simulink subsystem "ElectricalThermalSystem"  (R2024b)
settings: Solver=VariableStepAuto  StartTime=0.0  StopTime=10.0  RelTol=1e-3
undefined symbols (not defined in the file): EnvAirTemp, PlantThrEstCmpPwr, PlntThrAirBpt, PlntThrAirCond, PlntThrAirCp, PlntThrAirCpBpt, PlntThrAirPrand, PlntThrAirRho, PlntThrAirVisc, PlntThrBattDCFlwRatio, PlntThrBattJacLen, PlntThrChArea, PlntThrChDia, PlntThrCoolCond, PlntThrCoolCp, PlntThrCoolCpBpt, PlntThrCoolPrand, PlntThrCoolRho, PlntThrCoolVisc, PlntThrDCJacLen, PlntThrEMJacLen, PlntThrEstCOPLut, PlntThrEstDTLut, PlntThrHeaterMaxPwr, PlntThrPmpDisp, PlntThrPmpHeadP, PlntThrPmpMaxSpd, PlntThrPmpMechEff, PlntThrPmpVolEff, PlntThrRadAirArea, PlntThrRadAirDh, PlntThrRadFanAreaFlw, PlntThrRadFlwCoef, PlntThrRadGapHeight, PlntThrRadLength, PlntThrRadNTubes, PlntThrRadTubeDh, PlntThrRadTubeHeight, PlntThrRadWidth
libraries: autolibutils x45
(part 2 of 4)

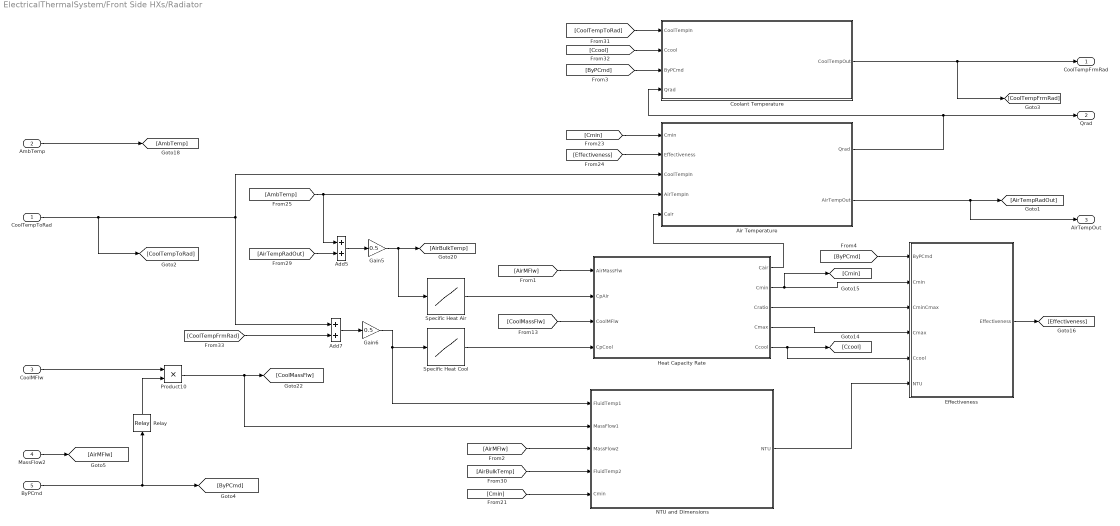
== system ElectricalThermalSystem/Front Side HXs/Radiator ==
  CoolTempToRad : Inport
  AmbTemp : Inport  Port=2
  CoolMFlw : Inport  Port=3
  MassFlow2 : Inport  Port=4
  ByPCmd : Inport  Port=5
  Add5 : Sum
  Add7 : Sum
  Air Temperature : Subsystem
      mask DialogControl DescTextVar Prompt: Air Temperature
      mask DialogControl ParameterGroupVar Prompt: Description
      mask DialogControl Control2 Prompt: Calculates the change in air temperature through the radiator and adds it to the inlet temperature to calculate the outlet temperature. In order to do that, the heat dissipated is calculated, using the effectiveness of the heat exchanger.
      mask DialogControl Control3 Prompt: Q = Effectiveness * Cmin * (Tcool - Tair)
      mask DialogControl Control4 Prompt: Where:
      mask DialogControl Control5 Prompt: Q: heat-flow rate
      mask DialogControl Control6 Prompt: Cmin: min(heat capacity rate air vs coolant)
      mask DialogControl Control7 Prompt: Heat capacity rate: heat capacity * fluid mass flow
      mask DialogControl Control8 Prompt: Tcool: coolant temperature (inlet)
      mask DialogControl Control9 Prompt: Tair: air temperature (inlet)
  Coolant Temperature : Subsystem
      mask DialogControl DescTextVar Prompt: Coolant Temperature
      mask DialogControl ParameterGroupVar Prompt: Description
      mask DialogControl Control2 Prompt: Calculates the change in coolant temperature through the radiator and adds it to the inlet temperature to calculate the outlet temperature.
      mask DialogControl Control3 Prompt: Q = Cool*(Tout-Tin)
      mask DialogControl Control4 Prompt: Where:
      mask DialogControl Control5 Prompt: Q: heat-flow rate
      mask DialogControl Control6 Prompt: Ccool (heat capacity rate) = mdot * Cp
      mask DialogControl Control7 Prompt: mdot: mass flow
      mask DialogControl Control8 Prompt: Cp: heat capacity
      mask DialogControl Control10 Prompt: Tout: temperature (outlet)
      mask DialogControl Control9 Prompt: Tin: temperature (inlet)
  Effectiveness : Subsystem
      mask DialogControl DescTextVar Prompt: Effectiveness
      mask DialogControl ParameterGroupVar Prompt: Description
      mask DialogControl Control2 Prompt: Effectiveness is calculated with NTU, according to the heat capacity rate ratio between the two fluids (air, coolant).
      mask DialogControl Control3 Prompt: If Cmax == Ccool: Effectiveness = (Cmax/Cmin)* (1-exp(-(Cmin/Cmax)*(1-exp(-NTU))))
      mask DialogControl Control4 Prompt: If Cmin == Ccool: Efectiveness = 1-exp((-Cmax/Cmin)*(1-exp(-Cmin/Cmax*NTU)))
      mask DialogControl Control5 Prompt: Where:
      mask DialogControl Control6 Prompt: Cmax: maximum heat capacity rate between the two fluids
      mask DialogControl Control7 Prompt: Cmin: minimum heat capacity rate between the two fluids
      mask DialogControl Control9 Prompt: Ccool: coolant heat capacity rate
      mask DialogControl Control8 Prompt: Heat capacity rate: heat capacity * fluid mass flow
  Gain5 : Gain  Gain=0.5
  Gain6 : Gain  Gain=0.5
  Heat Capacity Rate : Subsystem
      mask DialogControl DescTextVar Prompt: Heat Capacity Rate
      mask DialogControl ParameterGroupVar Prompt: Description
      mask DialogControl Control2 Prompt: Heat capacity rates (Cair, Ccool) are calculated for the two fluids in the heat exchanger, air and coolant.
      mask DialogControl Control3 Prompt: Cair and Ccool are used for NTU, temperature and effectiveness calculations.
      mask DialogControl Control4 Prompt: Heat capacity rate: heat capacity * fluid mass flow
  NTU and Dimensions : Subsystem  mask{NTubes=PlntThrRadNTubes, DhCool=PlntThrRadTubeDh, RadLen=PlntThrRadLength, RadWid=PlntThrRadWidth, DhAir=PlntThrRadAirDh, AcCool=PlntThrRadWidth*PlntThrRadTubeHeight, AcAir=PlntThrRadLength*PlntThrRadGapHeight*0.9}
      mask prompts: NTubes "Number of tubes, [-]"; DhCool "Hydraulic diameter coolant side, DhCool [m]"; RadLen "Radiator length, RadLen"; RadWid "Radiator width, RadWid"; DhAir "Hydraulic diameter air side, DhAir [m]"; AcCool "Cross-sectional area coolant side, AcCool [m^2]"; AcAir "Cross-sectional area air side, AcAir"
      mask TypeOptions NTubes: Constant/Value
      mask TypeOptions DhCool: Constant1/Value
      mask TypeOptions RadLen: Constant6/Value
      mask TypeOptions RadWid: Constant2/Value
      mask TypeOptions DhAir: Constant4/Value
      mask TypeOptions AcCool: Constant7/Value
      mask TypeOptions AcAir: Constant8/Value
      mask DialogControl DescTextVar Prompt: Number of Heat Transfer Units (NTU) and Radiator Dimensions
      mask DialogControl ParameterGroupVar Prompt: Description
      mask DialogControl Control1 Prompt: In heat exchangers NTU is a measure of heat transfer size.
      mask DialogControl Control3 Prompt: NTU = UA/Cmin
      mask DialogControl Control4 Prompt: Where:
      mask DialogControl Control5 Prompt: UA = 1/((1/HTCa*A)+(1/HTCc*A))
      mask DialogControl Control6 Prompt: Where:
      mask DialogControl Control7 Prompt: HTCa: convective heat transfer coefficient air side
      mask DialogControl Control8 Prompt: HTCc: convective heat transfer coefficient coolant side
      mask DialogControl Control9 Prompt: A: heat transfer area
      mask DialogControl Control10 Prompt: Cmin: min(heat capacity rate air vs coolant)
      mask DialogControl Control11 Prompt: Heat capacity rate: heat capacity * fluid mass flow
      mask DialogControl Container3 Prompt: Parameters
  Product10 : Product
  Relay : Relay  OnSwitchValue=0.5  OffSwitchValue=0.5  OnOutputValue=eps  OffOutputValue=1
  Specific Heat Air : Lookup_n-D  NumberOfTableDimensions=1  BreakpointsForDimension1=PlntThrAirCpBpt  Table=PlntThrAirCp  ExtrapMethod=Clip  UseLastTableValue=on  InternalRulePriority=Speed  RndMeth=Simplest
  Specific Heat Cool : Lookup_n-D  NumberOfTableDimensions=1  BreakpointsForDimension1=PlntThrCoolCpBpt  Table=PlntThrCoolCp  ExtrapMethod=Clip  UseLastTableValue=on  InternalRulePriority=Speed  RndMeth=Simplest
  CoolTempFrmRad : Outport
  Qrad : Outport  Port=2
  AirTempOut : Outport  Port=3
  wires:
  CoolTempToRad/1 -> Air Temperature/3(CoolTempIn), Add7/1, [CoolTempToRad]
  Gain6/1 -> NTU and Dimensions/1(FluidTemp1), Specific Heat Cool/1
  [AirBulkTemp] -> NTU and Dimensions/4(FluidTemp2)
  [CoolTempFrmRad] -> Add7/2
  CoolMFlw/1 -> Product10/1
  Product10/1 -> NTU and Dimensions/2(MassFlow1), [CoolMassFlw]
  [AmbTemp] -> Add5/1, Air Temperature/4(AirTempIn)
  ByPCmd/1 -> [ByPCmd], Relay/1
  [Cmin] -> NTU and Dimensions/5(Cmin)
  AmbTemp/1 -> [AmbTemp]
  [AirTempRadOut] -> Add5/2
  Add5/1 -> Gain5/1
  Gain5/1 -> Specific Heat Air/1, [AirBulkTemp]
  Relay/1 -> Product10/2
  Add7/1 -> Gain6/1
  MassFlow2/1 -> [AirMFlw]
  [AirMFlw] -> NTU and Dimensions/3(MassFlow2)
  Heat Capacity Rate/2(Cmin) -> Effectiveness/2(Cmin), [Cmin]
  [AirMFlw] -> Heat Capacity Rate/1(AirMassFlw)
  Specific Heat Air/1 -> Heat Capacity Rate/2(CpAir)
  [CoolMassFlw] -> Heat Capacity Rate/3(CoolMFlw)
  Specific Heat Cool/1 -> Heat Capacity Rate/4(CpCool)
  [ByPCmd] -> Effectiveness/1(ByPCmd)
  Heat Capacity Rate/3(Cratio) -> Effectiveness/3(CminCmax)
  Heat Capacity Rate/4(Cmax) -> Effectiveness/4(Cmax)
  Heat Capacity Rate/5(Ccool) -> Effectiveness/5(Ccool), [Ccool]
  NTU and Dimensions/1(NTU) -> Effectiveness/6(NTU)
  Effectiveness/1(Effectiveness) -> [Effectiveness]
  Coolant Temperature/1(CoolTempOut) -> CoolTempFrmRad/1, [CoolTempFrmRad]
  [CoolTempToRad] -> Coolant Temperature/1(CoolTempIn)
  [Ccool] -> Coolant Temperature/2(Ccool)
  Air Temperature/2(AirTempOut) -> AirTempOut/1, [AirTempRadOut]
  Air Temperature/1(Qrad) -> Coolant Temperature/4(Qrad), Qrad/1
  [Cmin] -> Air Temperature/1(Cmin)
  [Effectiveness] -> Air Temperature/2(Effectiveness)
  Heat Capacity Rate/1(Cair) -> Air Temperature/5(Cair)
  [ByPCmd] -> Coolant Temperature/3(ByPCmd)

== system ElectricalThermalSystem/Heater Battery DCDC Converter/Battery ==
  FluidTemp : Inport
  MassFlow : Inport  Port=2
  BattTemp : Inport  Port=3
  Constant3 : Constant  Value=JacHtArea  SampleTime=-1
  Constant6 : Constant  Value=JacDia  SampleTime=-1
  Constant7 : Constant  Value=JacArea  SampleTime=-1
  Constant8 : Constant  Value=JacLen  SampleTime=-1
  HTC Estimator Batt : Subsystem
      mask DialogControl Control1 Prompt: Convective Heat Transfer Coefficient (HTC) Estimator
      mask DialogControl Container2 Prompt: Description
      mask DialogControl Control2 Prompt: Assumes turbulent flow through a tube.
      mask DialogControl Control3 Prompt: The Nusselt number (NuD) is calculated with empirical formulas depending on 1/DoL.
      mask DialogControl Control4 Prompt: Where:
      mask DialogControl Control5 Prompt: DoL = hydraulic diameter / tube length
      mask DialogControl Control6 Prompt: When 1/DoL >= 400: NuD = 0.023*ReD^0.8*Pr^0.33
      mask DialogControl Control7 Prompt: Where:
      mask DialogControl Control8 Prompt: Pr: Prandtl number, out of 1D LUT depending on fluid temperature
      mask DialogControl Control9 Prompt: ReD: Reynolds number, calculated. ReD = mdot*hdia/(Ac*aVsc)
      mask DialogControl Control10 Prompt: Where:
      mask DialogControl Control11 Prompt: mdot: mass flow
      mask DialogControl Control12 Prompt: hdia: hydraulic diameter
      mask DialogControl Control13 Prompt: Ac: cross section area
      mask DialogControl Control14 Prompt: aVsc: absolute viscosity, out of 1D LUT depending on fluid temperature
      mask DialogControl Control15 Prompt: When 1/DoL < 400: NuD = 0.36*ReD^0.8*Pr^0.33*DoL^0.055
      mask DialogControl Control16 Prompt: Finally, HTC = k*NuD/hdia
      mask DialogControl Control17 Prompt: Where:
      mask DialogControl Control18 Prompt: k: thermal conductivity, out of 1D LUT depending on fluid temperature
  Heat-flow Rate : Subsystem
  Qbatt : Outport
  wires:
  Constant7/1 -> HTC Estimator Batt/3(CrossA)
  Constant8/1 -> HTC Estimator Batt/5(TubLen)
  Constant6/1 -> HTC Estimator Batt/4(HydDia)
  MassFlow/1 -> HTC Estimator Batt/2(MassFlow)
  HTC Estimator Batt/1(HTC) -> Heat-flow Rate/1(HTC)
  Constant3/1 -> Heat-flow Rate/2(JacHtArea)
  BattTemp/1 -> Heat-flow Rate/3(BattTemp)
  FluidTemp/1 -> Heat-flow Rate/4(CoolBlkTemp), HTC Estimator Batt/1(FluidTemp)
  Heat-flow Rate/1(Qbatt) -> Qbatt/1

== system ElectricalThermalSystem/Heater Battery DCDC Converter/Battery Heater ==
  HeaterCmd : Inport
  BattCoolMFlw : Inport  Port=2
  CoolTempIn : Inport  Port=3
  Add : Sum
  Add4 : Sum
  Divide1 : Product  Inputs=*/
  Gain4 : Gain  Gain=0.5
  LPF with IC3 : Subsystem  mask{wc=10, InitCond=EnvAirTemp, dataType=off}
      mask prompts: wc "Cutoff frequency, wc [rad/s]"; InitCond "Initial condition, InitCond [same as u]"; dataType "Enforce same input data type"
      mask TypeOptions wc: Cont LPF IC/wc
      mask TypeOptions InitCond: Initial Condition/Value
      mask TypeOptions dataType: Cont LPF IC/dataType
  Max Heat : Gain  Gain=HtPwr
  Product : Product
  Specific Heat1 : Lookup_n-D  NumberOfTableDimensions=1  BreakpointsForDimension1=PlntThrCoolCpBpt  Table=PlntThrCoolCp  ExtrapMethod=Clip  UseLastTableValue=on  InternalRulePriority=Speed  RndMeth=Simplest
  div0protect - abs poly1 : autolibutils/div0protect - abs poly  thresh=.001  aMode=1
  Qheater : Outport
  CoolBattTemp : Outport  Port=2
  wires:
  Gain4/1 -> Specific Heat1/1
  Divide1/1 -> Add/1
  Specific Heat1/1 -> Product/2
  Product/1 -> div0protect - abs poly1/1
  CoolTempIn/1 -> Add/2, Add4/2
  Add4/1 -> Gain4/1
  Max Heat/1 -> Qheater/1, Divide1/1
  div0protect - abs poly1/1 -> Divide1/2
  BattCoolMFlw/1 -> Product/1
  [CoolBattTempIn] -> Add4/1
  HeaterCmd/1 -> Max Heat/1
  Add/1 -> LPF with IC3/1(u)
  LPF with IC3/1(y) -> [CoolBattTempIn], CoolBattTemp/1

== system ElectricalThermalSystem/Heater Battery DCDC Converter/Coolant Mass Flow Distribution ==
  CoolMFlw : Inport
  Gain2 : Gain  Gain=MFlwRt
  Minus1 : Sum  Inputs=+-
  DCCoolMFlw : Outport
  BattCoolMFlw : Outport  Port=2
  wires:
  Gain2/1 -> BattCoolMFlw/1, Minus1/2
  CoolMFlw/1 -> Minus1/1, Gain2/1
  Minus1/1 -> DCCoolMFlw/1

== system ElectricalThermalSystem/Heater Battery DCDC Converter/Coolant Temperature ==
  Qsum : Inport
  CoolMFlw : Inport  Port=2
  CoolBlkTemp : Inport  Port=3
  Divide : Product  Inputs=*/
  Product3 : Product
  Specific Heat : Lookup_n-D  NumberOfTableDimensions=1  BreakpointsForDimension1=PlntThrCoolCpBpt  Table=PlntThrCoolCp  ExtrapMethod=Clip  UseLastTableValue=on  InternalRulePriority=Speed  RndMeth=Simplest
  div0protect - abs poly4 : autolibutils/div0protect - abs poly  thresh=.001  aMode=1
  DeltaTemp : Outport
  wires:
  Specific Heat/1 -> Product3/2
  Product3/1 -> div0protect - abs poly4/1
  div0protect - abs poly4/1 -> Divide/2
  CoolMFlw/1 -> Product3/1
  Qsum/1 -> Divide/1
  CoolBlkTemp/1 -> Specific Heat/1
  Divide/1 -> DeltaTemp/1

== system ElectricalThermalSystem/Heater Battery DCDC Converter/DC-DC Converter ==
  FluidTemp : Inport
  MassFlow : Inport  Port=2
  PwrETemp : Inport  Port=3
  Constant : Constant  Value=JacDia  SampleTime=-1
  Constant2 : Constant  Value=JacHtArea  SampleTime=-1
  Constant4 : Constant  Value=JacArea  SampleTime=-1
  Constant5 : Constant  Value=JacLen  SampleTime=-1
  HTC Estimator DCDC : Subsystem
      mask DialogControl Control1 Prompt: Convective Heat Transfer Coefficient (HTC) Estimator
      mask DialogControl Container2 Prompt: Description
      mask DialogControl Control2 Prompt: Assumes turbulent flow through a tube.
      mask DialogControl Control3 Prompt: The Nusselt number (NuD) is calculated with empirical formulas depending on 1/DoL.
      mask DialogControl Control4 Prompt: Where:
      mask DialogControl Control5 Prompt: DoL = hydraulic diameter / tube length
      mask DialogControl Control6 Prompt: When 1/DoL >= 400: NuD = 0.023*ReD^0.8*Pr^0.33
      mask DialogControl Control7 Prompt: Where:
      mask DialogControl Control8 Prompt: Pr: Prandtl number, out of 1D LUT depending on fluid temperature
      mask DialogControl Control9 Prompt: ReD: Reynolds number, calculated. ReD = mdot*hdia/(Ac*aVsc)
      mask DialogControl Control10 Prompt: Where:
      mask DialogControl Control11 Prompt: mdot: mass flow
      mask DialogControl Control12 Prompt: hdia: hydraulic diameter
      mask DialogControl Control13 Prompt: Ac: cross section area
      mask DialogControl Control14 Prompt: aVsc: absolute viscosity, out of 1D LUT depending on fluid temperature
      mask DialogControl Control15 Prompt: When 1/DoL < 400: NuD = 0.36*ReD^0.8*Pr^0.33*DoL^0.055
      mask DialogControl Control16 Prompt: Finally, HTC = k*NuD/hdia
      mask DialogControl Control17 Prompt: Where:
      mask DialogControl Control18 Prompt: k: thermal conductivity, out of 1D LUT depending on fluid temperature
  Heat-flow Rate : Subsystem
  Qpwre : Outport
  wires:
  Constant/1 -> HTC Estimator DCDC/4(HydDia)
  Constant5/1 -> HTC Estimator DCDC/5(TubLen)
  Constant4/1 -> HTC Estimator DCDC/3(CrossA)
  MassFlow/1 -> HTC Estimator DCDC/2(MassFlow)
  HTC Estimator DCDC/1(HTC) -> Heat-flow Rate/1(HTC)
  PwrETemp/1 -> Heat-flow Rate/2(PwrETemp)
  Constant2/1 -> Heat-flow Rate/3(JacArea)
  FluidTemp/1 -> Heat-flow Rate/4(CoolBlkTemp), HTC Estimator DCDC/1(FluidTemp)
  Heat-flow Rate/1(Qpwre) -> Qpwre/1

== system ElectricalThermalSystem/Heater Battery DCDC Converter/LPF with IC1 ==
  u : Inport
  Cont LPF IC : autolibutils/Cont LPF IC  wc=wc  aMode=1  dataType=off
  Initial Condition : Constant  Value=InitCond  SampleTime=-1
  y : Outport
  wires:
  Initial Condition/1 -> Cont LPF IC/2
  u/1 -> Cont LPF IC/1
  Cont LPF IC/1 -> y/1

== system ElectricalThermalSystem/Heater Battery DCDC Converter/LPF with IC2 ==
  u : Inport
  Cont LPF IC : autolibutils/Cont LPF IC  wc=wc  aMode=1  dataType=off
  Initial Condition : Constant  Value=InitCond  SampleTime=-1
  y : Outport
  wires:
  Initial Condition/1 -> Cont LPF IC/2
  u/1 -> Cont LPF IC/1
  Cont LPF IC/1 -> y/1

== system ElectricalThermalSystem/Heater Battery DCDC Converter/LPF with IC4 ==
  u : Inport
  Cont LPF IC : autolibutils/Cont LPF IC  wc=wc  aMode=1  dataType=off
  Initial Condition : Constant  Value=InitCond  SampleTime=-1
  y : Outport
  wires:
  Initial Condition/1 -> Cont LPF IC/2
  u/1 -> Cont LPF IC/1
  Cont LPF IC/1 -> y/1

== system ElectricalThermalSystem/Motor/FourEMs ==
  EMTemp : Inport
  CoolMFlow : Inport  Port=2
  CoolTempIn : Inport  Port=3
  EM1 : Subsystem  mask{JacArea=PlntThrChArea, JacDia=PlntThrChDia, JacLen=PlntThrEMJacLen, JacHtArea=PlntThrEMJacLen*pi*PlntThrChDia}
      mask prompts: JacArea "Jacket cross section area, JacArea [m^2]"; JacDia "Jacket hydraulic diameter, JacDia [m]"; JacLen "Jacket length, JacLen [m]"; JacHtArea "Jacket heat transfer area, JacHtArea [m^2]"
      mask TypeOptions JacArea: Constant2/Value
      mask TypeOptions JacDia: Constant1/Value
      mask TypeOptions JacLen: Constant3/Value
      mask TypeOptions JacHtArea: Constant/Value
      mask DialogControl DescTextVar Prompt: Electric Machine Heat Transfer
      mask DialogControl ParameterGroupVar Prompt: Description
      mask DialogControl Control2 Prompt: The cooling of the electric machine is estimated with a cooling jacket.
      mask DialogControl Container3 Prompt: Parameters
  EM2 : Subsystem  mask{JacArea=PlntThrChArea, JacDia=PlntThrChDia, JacLen=PlntThrEMJacLen, JacHtArea=PlntThrEMJacLen*pi*PlntThrChDia}
      mask prompts: JacArea "Jacket cross section area, JacArea [m^2]"; JacDia "Jacket hydraulic diameter, JacDia [m]"; JacLen "Jacket length, JacLen [m]"; JacHtArea "Jacket heat transfer area, JacHtArea [m^2]"
      mask TypeOptions JacArea: Constant2/Value
      mask TypeOptions JacDia: Constant1/Value
      mask TypeOptions JacLen: Constant3/Value
      mask TypeOptions JacHtArea: Constant/Value
      mask DialogControl DescTextVar Prompt: Electric Machine Heat Transfer
      mask DialogControl ParameterGroupVar Prompt: Description
      mask DialogControl Control2 Prompt: The cooling of the electric machine is estimated with a cooling jacket.
      mask DialogControl Container3 Prompt: Parameters
  EM3 : Subsystem  mask{JacArea=PlntThrChArea, JacDia=PlntThrChDia, JacLen=PlntThrEMJacLen, JacHtArea=PlntThrEMJacLen*pi*PlntThrChDia}
      mask prompts: JacArea "Jacket cross section area, JacArea [m^2]"; JacDia "Jacket hydraulic diameter, JacDia [m]"; JacLen "Jacket length, JacLen [m]"; JacHtArea "Jacket heat transfer area, JacHtArea [m^2]"
      mask TypeOptions JacArea: Constant2/Value
      mask TypeOptions JacDia: Constant1/Value
      mask TypeOptions JacLen: Constant3/Value
      mask TypeOptions JacHtArea: Constant/Value
      mask DialogControl DescTextVar Prompt: Electric Machine Heat Transfer
      mask DialogControl ParameterGroupVar Prompt: Description
      mask DialogControl Control2 Prompt: The cooling of the electric machine is estimated with a cooling jacket.
      mask DialogControl Container3 Prompt: Parameters
  EM4 : Subsystem  mask{JacArea=PlntThrChArea, JacDia=PlntThrChDia, JacLen=PlntThrEMJacLen, JacHtArea=PlntThrEMJacLen*pi*PlntThrChDia}
      mask prompts: JacArea "Jacket cross section area, JacArea [m^2]"; JacDia "Jacket hydraulic diameter, JacDia [m]"; JacLen "Jacket length, JacLen [m]"; JacHtArea "Jacket heat transfer area, JacHtArea [m^2]"
      mask TypeOptions JacArea: Constant2/Value
      mask TypeOptions JacDia: Constant1/Value
      mask TypeOptions JacLen: Constant3/Value
      mask TypeOptions JacHtArea: Constant/Value
      mask DialogControl DescTextVar Prompt: Electric Machine Heat Transfer
      mask DialogControl ParameterGroupVar Prompt: Description
      mask DialogControl Control2 Prompt: The cooling of the electric machine is estimated with a cooling jacket.
      mask DialogControl Container3 Prompt: Parameters
  Max of Elements : MinMax  Function=max
  Vector Concatenate : Concatenate  NumInputs=4
  Bus Element Out3 : Outport  PortName=Info  Element=Qem
  Bus Element Out1 : Outport  PortName=Info  Element=CoolTempOut
  Bus Element Out4 : Outport  PortName=Info  Element=MotorTemp
  wires:
  CoolMFlow/1 -> [MassFlow], EM1/2(CoolMFlow)
  CoolTempIn/1 -> EM1/1(CoolTempIn)
  EMTemp/1 -> Max of Elements/1, [EMTemp], EM1/3(EMTemp)
  EM1/2(CoolTempOut) -> EM2/1(CoolTempIn)
  EM1/1(Qem) -> Vector Concatenate/1
  EM2/1(Qem) -> Vector Concatenate/2
  Vector Concatenate/1 -> Bus Element Out3/1
  Max of Elements/1 -> Bus Element Out4/1
  [MassFlow] -> EM2/2(CoolMFlow)
  [EMTemp] -> EM2/3(EMTemp)
  EM2/2(CoolTempOut) -> EM3/1(CoolTempIn)
  [MassFlow] -> EM3/2(CoolMFlow)
  [EMTemp] -> EM3/3(EMTemp)
  EM3/1(Qem) -> Vector Concatenate/3
  EM4/2(CoolTempOut) -> Bus Element Out1/1
  EM3/2(CoolTempOut) -> EM4/1(CoolTempIn)
  [MassFlow] -> EM4/2(CoolMFlow)
  [EMTemp] -> EM4/3(EMTemp)
  EM4/1(Qem) -> Vector Concatenate/4

== system ElectricalThermalSystem/Motor/OneEM ==
  EMTemp : Inport
  CoolMFlow : Inport  Port=2
  CoolTempIn : Inport  Port=3
  EM1 : Subsystem  mask{JacArea=PlntThrChArea, JacDia=PlntThrChDia, JacLen=PlntThrEMJacLen, JacHtArea=PlntThrEMJacLen*pi*PlntThrChDia}
      mask prompts: JacArea "Jacket cross section area, JacArea [m^2]"; JacDia "Jacket hydraulic diameter, JacDia [m]"; JacLen "Jacket length, JacLen [m]"; JacHtArea "Jacket heat transfer area, JacHtArea [m^2]"
      mask TypeOptions JacArea: Constant2/Value
      mask TypeOptions JacDia: Constant1/Value
      mask TypeOptions JacLen: Constant3/Value
      mask TypeOptions JacHtArea: Constant/Value
      mask DialogControl DescTextVar Prompt: Electric Machine Heat Transfer
      mask DialogControl ParameterGroupVar Prompt: Description
      mask DialogControl Control2 Prompt: The cooling of the electric machine is estimated with a cooling jacket.
      mask DialogControl Container3 Prompt: Parameters
  Bus Element Out3 : Outport  PortName=Info  Element=Qem
  Bus Element Out1 : Outport  PortName=Info  Element=CoolTempOut
  Bus Element Out4 : Outport  PortName=Info  Element=MotorTemp
  wires:
  CoolMFlow/1 -> EM1/1(MassFlow)
  CoolTempIn/1 -> EM1/2(CoolTempIn)
  EM1/1(Qem) -> Bus Element Out3/1
  EMTemp/1 -> Bus Element Out4/1, EM1/3(EMTemp)
  EM1/2(CoolTempOut) -> Bus Element Out1/1

== system ElectricalThermalSystem/Motor/ThreeEMs ==
  EMTemp : Inport
  CoolMFlow : Inport  Port=2
  CoolTempIn : Inport  Port=3
  EM1 : Subsystem  mask{JacArea=PlntThrChArea, JacDia=PlntThrChDia, JacLen=PlntThrEMJacLen, JacHtArea=PlntThrEMJacLen*pi*PlntThrChDia}
      mask prompts: JacArea "Jacket cross section area, JacArea [m^2]"; JacDia "Jacket hydraulic diameter, JacDia [m]"; JacLen "Jacket length, JacLen [m]"; JacHtArea "Jacket heat transfer area, JacHtArea [m^2]"
      mask TypeOptions JacArea: Constant2/Value
      mask TypeOptions JacDia: Constant1/Value
      mask TypeOptions JacLen: Constant3/Value
      mask TypeOptions JacHtArea: Constant/Value
      mask DialogControl DescTextVar Prompt: Electric Machine Heat Transfer
      mask DialogControl ParameterGroupVar Prompt: Description
      mask DialogControl Control2 Prompt: The cooling of the electric machine is estimated with a cooling jacket.
      mask DialogControl Container3 Prompt: Parameters
  EM2 : Subsystem  mask{JacArea=PlntThrChArea, JacDia=PlntThrChDia, JacLen=PlntThrEMJacLen, JacHtArea=PlntThrEMJacLen*pi*PlntThrChDia}
      mask prompts: JacArea "Jacket cross section area, JacArea [m^2]"; JacDia "Jacket hydraulic diameter, JacDia [m]"; JacLen "Jacket length, JacLen [m]"; JacHtArea "Jacket heat transfer area, JacHtArea [m^2]"
      mask TypeOptions JacArea: Constant2/Value
      mask TypeOptions JacDia: Constant1/Value
      mask TypeOptions JacLen: Constant3/Value
      mask TypeOptions JacHtArea: Constant/Value
      mask DialogControl DescTextVar Prompt: Electric Machine Heat Transfer
      mask DialogControl ParameterGroupVar Prompt: Description
      mask DialogControl Control2 Prompt: The cooling of the electric machine is estimated with a cooling jacket.
      mask DialogControl Container3 Prompt: Parameters
  EM3 : Subsystem  mask{JacArea=PlntThrChArea, JacDia=PlntThrChDia, JacLen=PlntThrEMJacLen, JacHtArea=PlntThrEMJacLen*pi*PlntThrChDia}
      mask prompts: JacArea "Jacket cross section area, JacArea [m^2]"; JacDia "Jacket hydraulic diameter, JacDia [m]"; JacLen "Jacket length, JacLen [m]"; JacHtArea "Jacket heat transfer area, JacHtArea [m^2]"
      mask TypeOptions JacArea: Constant2/Value
      mask TypeOptions JacDia: Constant1/Value
      mask TypeOptions JacLen: Constant3/Value
      mask TypeOptions JacHtArea: Constant/Value
      mask DialogControl DescTextVar Prompt: Electric Machine Heat Transfer
      mask DialogControl ParameterGroupVar Prompt: Description
      mask DialogControl Control2 Prompt: The cooling of the electric machine is estimated with a cooling jacket.
      mask DialogControl Container3 Prompt: Parameters
  Max of Elements : MinMax  Function=max
  Vector Concatenate : Concatenate  NumInputs=3
  Bus Element Out3 : Outport  PortName=Info  Element=Qem
  Bus Element Out1 : Outport  PortName=Info  Element=CoolTempOut
  Bus Element Out4 : Outport  PortName=Info  Element=MotorTemp
  wires:
  CoolMFlow/1 -> [MassFlow], EM1/2(CoolMFlow)
  CoolTempIn/1 -> EM1/1(CoolTempIn)
  EMTemp/1 -> Max of Elements/1, [EMTemp], EM1/3(EMTemp)
  EM1/2(CoolTempOut) -> EM2/1(CoolTempIn)
  EM1/1(Qem) -> Vector Concatenate/1
  EM2/1(Qem) -> Vector Concatenate/2
  Vector Concatenate/1 -> Bus Element Out3/1
  Max of Elements/1 -> Bus Element Out4/1
  [MassFlow] -> EM2/2(CoolMFlow)
  [EMTemp] -> EM2/3(EMTemp)
  EM3/2(CoolTempOut) -> Bus Element Out1/1
  EM2/2(CoolTempOut) -> EM3/1(CoolTempIn)
  [MassFlow] -> EM3/2(CoolMFlow)
  [EMTemp] -> EM3/3(EMTemp)
  EM3/1(Qem) -> Vector Concatenate/3

== system ElectricalThermalSystem/Motor/TwoEMs ==
  EMTemp : Inport
  CoolMFlow : Inport  Port=2
  CoolTempIn : Inport  Port=3
  EM1 : Subsystem  mask{JacArea=PlntThrChArea, JacDia=PlntThrChDia, JacLen=PlntThrEMJacLen, JacHtArea=PlntThrEMJacLen*pi*PlntThrChDia}
      mask prompts: JacArea "Jacket cross section area, JacArea [m^2]"; JacDia "Jacket hydraulic diameter, JacDia [m]"; JacLen "Jacket length, JacLen [m]"; JacHtArea "Jacket heat transfer area, JacHtArea [m^2]"
      mask TypeOptions JacArea: Constant2/Value
      mask TypeOptions JacDia: Constant1/Value
      mask TypeOptions JacLen: Constant3/Value
      mask TypeOptions JacHtArea: Constant/Value
      mask DialogControl DescTextVar Prompt: Electric Machine Heat Transfer
      mask DialogControl ParameterGroupVar Prompt: Description
      mask DialogControl Control2 Prompt: The cooling of the electric machine is estimated with a cooling jacket.
      mask DialogControl Container3 Prompt: Parameters
  EM2 : Subsystem  mask{JacArea=PlntThrChArea, JacDia=PlntThrChDia, JacLen=PlntThrEMJacLen, JacHtArea=PlntThrEMJacLen*pi*PlntThrChDia}
      mask prompts: JacArea "Jacket cross section area, JacArea [m^2]"; JacDia "Jacket hydraulic diameter, JacDia [m]"; JacLen "Jacket length, JacLen [m]"; JacHtArea "Jacket heat transfer area, JacHtArea [m^2]"
      mask TypeOptions JacArea: Constant2/Value
      mask TypeOptions JacDia: Constant1/Value
      mask TypeOptions JacLen: Constant3/Value
      mask TypeOptions JacHtArea: Constant/Value
      mask DialogControl DescTextVar Prompt: Electric Machine Heat Transfer
      mask DialogControl ParameterGroupVar Prompt: Description
      mask DialogControl Control2 Prompt: The cooling of the electric machine is estimated with a cooling jacket.
      mask DialogControl Container3 Prompt: Parameters
  Max of Elements : MinMax  Function=max
  Vector Concatenate : Concatenate
  Bus Element Out3 : Outport  PortName=Info  Element=Qem
  Bus Element Out1 : Outport  PortName=Info  Element=CoolTempOut
  Bus Element Out4 : Outport  PortName=Info  Element=MotorTemp
  wires:
  CoolMFlow/1 -> [MassFlow], EM1/2(CoolMFlow)
  CoolTempIn/1 -> EM1/1(CoolTempIn)
  EMTemp/1 -> Max of Elements/1, [EMTemp], EM1/3(EMTemp)
  EM1/2(CoolTempOut) -> EM2/1(CoolTempIn)
  EM2/2(CoolTempOut) -> Bus Element Out1/1
  EM1/1(Qem) -> Vector Concatenate/1
  EM2/1(Qem) -> Vector Concatenate/2
  Vector Concatenate/1 -> Bus Element Out3/1
  Max of Elements/1 -> Bus Element Out4/1
  [MassFlow] -> EM2/2(CoolMFlow)
  [EMTemp] -> EM2/3(EMTemp)

== system ElectricalThermalSystem/Motor Pump/LPF with IC1 ==
  u : Inport
  Cont LPF IC : autolibutils/Cont LPF IC  wc=wc  aMode=1  dataType=off
  Initial Condition : Constant  Value=InitCond  SampleTime=-1
  y : Outport
  wires:
  Initial Condition/1 -> Cont LPF IC/2
  u/1 -> Cont LPF IC/1
  Cont LPF IC/1 -> y/1

== system ElectricalThermalSystem/Refrigeration Loop/Chiller Coolant Temperature ==
  Qchiller : Inport
  CoolTempOut : Inport  Port=2
  CoolTempIn : Inport  Port=3
  CoolMFlw : Inport  Port=4
  ByPCmd : Inport  Port=5
  Add : Sum
  Divide : Product  Inputs=*/
  Gain1 : Gain  Gain=0.5
  LPF with IC3 : Subsystem  mask{wc=10, InitCond=EnvAirTemp, dataType=off}
      mask prompts: wc "Cutoff frequency, wc [rad/s]"; InitCond "Initial condition, InitCond [same as u]"; dataType "Enforce same input data type"
      mask TypeOptions wc: Cont LPF IC/wc
      mask TypeOptions InitCond: Initial Condition/Value
      mask TypeOptions dataType: Cont LPF IC/dataType
  Minus : Sum
  Product : Product
  Specific Heat : Lookup_n-D  NumberOfTableDimensions=1  BreakpointsForDimension1=PlntThrCoolCpBpt  Table=PlntThrCoolCp  ExtrapMethod=Clip  UseLastTableValue=on  InternalRulePriority=Speed  RndMeth=Simplest
  Switch6 : Switch  Criteria=u2 > Threshold  Threshold=0.5  SaturateOnIntegerOverflow=off  InputSameDT=off
  div0protect - abs poly2 : autolibutils/div0protect - abs poly  thresh=.001  aMode=1
  CoolTOut : Outport
  wires:
  Divide/1 -> Minus/2
  CoolTempIn/1 -> Add/2, [CoolTempIn]
  Add/1 -> Gain1/1
  Minus/1 -> LPF with IC3/1(u)
  LPF with IC3/1(y) -> Switch6/3
  [CoolTempIn] -> Minus/1, Switch6/1
  div0protect - abs poly2/1 -> Divide/2
  Gain1/1 -> Specific Heat/1
  ByPCmd/1 -> Switch6/2
  Specific Heat/1 -> Product/1
  Product/1 -> div0protect - abs poly2/1
  CoolTempOut/1 -> Add/1
  Switch6/1 -> CoolTOut/1
  Qchiller/1 -> Divide/1
  CoolMFlw/1 -> Product/2

== system ElectricalThermalSystem/Refrigeration Loop/Chiller Pressure ==
  CoolTempIn : Inport
  CoolTempOut : Inport  Port=2
  1-D Lookup Table2 : Lookup_n-D  NumberOfTableDimensions=1  BreakpointsForDimension1=[0 1 3 7]  Table=[0.65 0.45 0.3 0.3]  ExtrapMethod=Clip  UseLastTableValue=on  InternalRulePriority=Speed  RndMeth=Simplest
  Subtract3 : Sum  Inputs=+-
  ChlrPress : Outport
  wires:
  Subtract3/1 -> 1-D Lookup Table2/1
  CoolTempIn/1 -> Subtract3/1
  CoolTempOut/1 -> Subtract3/2
  1-D Lookup Table2/1 -> ChlrPress/1

== system ElectricalThermalSystem/Refrigeration Loop/Condenser Pressure ==
  AirTempOut : Inport
  AirTempIn : Inport  Port=2
  1-D Lookup Table1 : Lookup_n-D  NumberOfTableDimensions=1  BreakpointsForDimension1=[0 4.5 10 13 20]  Table=[1.3 1.3 1.53 1.62 1.7]  ExtrapMethod=Clip  UseLastTableValue=on  InternalRulePriority=Speed  RndMeth=Simplest
  Subtract1 : Sum  Inputs=+-
  CondPress : Outport
  wires:
  Subtract1/1 -> 1-D Lookup Table1/1
  AirTempOut/1 -> Subtract1/1
  AirTempIn/1 -> Subtract1/2
  1-D Lookup Table1/1 -> CondPress/1

== system ElectricalThermalSystem/Refrigeration Loop/Heat-flow Rate and Power ==
  AmbTemp : Inport
  CoolTempIn : Inport  Port=2
  CmpCmd : Inport  Port=3
  1-D Lookup Table : Lookup_n-D  NumberOfTableDimensions=1  BreakpointsForDimension1=PlntThrEstDTLut  Table=PlntThrEstCOPLut  ExtrapMethod=Clip  InternalRulePriority=Speed  RndMeth=Simplest
  Add1 : Sum
  Gain : Gain  Gain=-1
  LPF with IC1 : Subsystem  mask{wc=0.2, InitCond=0, dataType=off}
      mask prompts: wc "Cutoff frequency, wc [rad/s]"; InitCond "Initial condition, InitCond [same as u]"; dataType "Enforce same input data type"
      mask TypeOptions wc: Cont LPF IC/wc
      mask TypeOptions InitCond: Initial Condition/Value
      mask TypeOptions dataType: Cont LPF IC/dataType
  Power Chiller : Product
  Power Comp : Gain  Gain=PlantThrEstCmpPwr
  Signal Specification : SignalSpecification  Unit=kW
  Signal Specification1 : SignalSpecification  Unit=watt
  Subtract : Sum  Inputs=+-
  Unit Conversion : UnitConversion
  Qcond : Outport
  CmpPwr : Outport  Port=2
  Qchiller : Outport  Port=3
  wires:
  Unit Conversion/1 -> Signal Specification1/1
  CoolTempIn/1 -> Subtract/2
  1-D Lookup Table/1 -> Power Chiller/1
  LPF with IC1/1(y) -> Power Comp/1
  [CmpPwr] -> Add1/1
  Subtract/1 -> 1-D Lookup Table/1
  Power Chiller/1 -> Add1/2, Gain/1
  Signal Specification/1 -> Unit Conversion/1
  Power Comp/1 -> Signal Specification/1
  Signal Specification1/1 -> CmpPwr/1, [CmpPwr], Power Chiller/2
  AmbTemp/1 -> Subtract/1
  Add1/1 -> Qcond/1
  Gain/1 -> Qchiller/1
  CmpCmd/1 -> LPF with IC1/1(u)

== system ElectricalThermalSystem/Front Side HXs/Condenser/LPF with IC2 ==
  u : Inport
  Cont LPF IC : autolibutils/Cont LPF IC  wc=wc  aMode=1  dataType=off
  Initial Condition : Constant  Value=InitCond  SampleTime=-1
  y : Outport
  wires:
  Initial Condition/1 -> Cont LPF IC/2
  u/1 -> Cont LPF IC/1
  Cont LPF IC/1 -> y/1

== system ElectricalThermalSystem/Front Side HXs/Radiator/Air Temperature ==
  Cmin : Inport
  Effectiveness : Inport  Port=2
  CoolTempIn : Inport  Port=3
  AirTempIn : Inport  Port=4
  Cair : Inport  Port=5
  Add4 : Sum
  LPF with IC1 : Subsystem  mask{wc=10, InitCond=EnvAirTemp, dataType=off}
      mask prompts: wc "Cutoff frequency, wc [rad/s]"; InitCond "Initial condition, InitCond [same as u]"; dataType "Enforce same input data type"
      mask TypeOptions wc: Cont LPF IC/wc
      mask TypeOptions InitCond: Initial Condition/Value
      mask TypeOptions dataType: Cont LPF IC/dataType
  Product3 : Product  Inputs=3
  Product5 : Product  Inputs=*/
  Saturation1 : Saturate  UpperLimit=inf  LowerLimit=173.15
  Subtract : Sum  Inputs=+-
  div0protect - abs poly1 : autolibutils/div0protect - abs poly  thresh=.001  aMode=1
  Qrad : Outport
  AirTempOut : Outport  Port=2
  wires:
  Subtract/1 -> Product3/3
  Cair/1 -> div0protect - abs poly1/1
  Add4/1 -> Saturation1/1
  Saturation1/1 -> LPF with IC1/1(u)
  div0protect - abs poly1/1 -> Product5/2
  Product3/1 -> Qrad/1, Product5/1
  LPF with IC1/1(y) -> AirTempOut/1
  Product5/1 -> Add4/2
  Cmin/1 -> Product3/1
  CoolTempIn/1 -> Subtract/1
  Effectiveness/1 -> Product3/2
  AirTempIn/1 -> [AirTempIn], Subtract/2
  [AirTempIn] -> Add4/1

== system ElectricalThermalSystem/Front Side HXs/Radiator/Coolant Temperature ==
  CoolTempIn : Inport
  Ccool : Inport  Port=2
  ByPCmd : Inport  Port=3
  Qrad : Inport  Port=4
  Add6 : Sum  Inputs=+-
  LPF Temperature : Subsystem  mask{wc=1, InitCond=EnvAirTemp, dataType=off}
      mask prompts: wc "Cutoff frequency, wc [rad/s]"; InitCond "Initial condition, InitCond [same as u]"; dataType "Enforce same input data type"
      mask TypeOptions wc: Cont LPF IC/wc
      mask TypeOptions InitCond: Initial Condition/Value
      mask TypeOptions dataType: Cont LPF IC/dataType
  Product6 : Product  Inputs=*/
  Saturation : Saturate  UpperLimit=inf  LowerLimit=173.15
  Switch5 : Switch  Criteria=u2 > Threshold  Threshold=0.5  SaturateOnIntegerOverflow=off  InputSameDT=off
  div0protect - abs poly : autolibutils/div0protect - abs poly  thresh=.001  aMode=1
  CoolTempOut : Outport
  wires:
  ByPCmd/1 -> Switch5/2
  Add6/1 -> Saturation/1
  Switch5/1 -> LPF Temperature/1(u)
  LPF Temperature/1(y) -> CoolTempOut/1
  Product6/1 -> Add6/2
  CoolTempIn/1 -> Add6/1, Switch5/1
  div0protect - abs poly/1 -> Product6/2
  Saturation/1 -> Switch5/3
  Qrad/1 -> Product6/1
  Ccool/1 -> div0protect - abs poly/1

== system ElectricalThermalSystem/Front Side HXs/Radiator/Effectiveness ==
  ByPCmd : Inport
  Cmin : Inport  Port=2
  CminCmax : Inport  Port=3
  Cmax : Inport  Port=4
  Ccool : Inport  Port=5
  NTU : Inport  Port=6
  Constant5 : Constant  SampleTime=-1
  Constant9 : Constant  Value=0  SampleTime=-1
  Effectiveness Calc : Fcn  Expr=(u(3)==u(5))*(1/u(2))*(1-exp(-u(2)*(1-exp(-u(4)))))+(u(1)==u(5))*(1-exp((-1/u(2))*(1-exp(-u(2)*u(4)))))
  Product2 : Product
  Switch1 : Switch  Criteria=u2 > Threshold  Threshold=0.5  SaturateOnIntegerOverflow=off  InputSameDT=off
  Vector Concatenate : Concatenate  NumInputs=5
  div0protect - abs poly5 : autolibutils/div0protect - abs poly  thresh=.001  aMode=1
  Effectiveness : Outport
  wires:
  Switch1/1 -> Product2/1
  Constant5/1 -> Switch1/3
  Constant9/1 -> Switch1/1
  Product2/1 -> Effectiveness/1
  Effectiveness Calc/1 -> Product2/2
  Cmax/1 -> Vector Concatenate/3
  Vector Concatenate/1 -> Effectiveness Calc/1
  Cmin/1 -> Vector Concatenate/1
  Ccool/1 -> Vector Concatenate/5
  ByPCmd/1 -> Switch1/2
  NTU/1 -> Vector Concatenate/4
  div0protect - abs poly5/1 -> Vector Concatenate/2
  CminCmax/1 -> div0protect - abs poly5/1

== system ElectricalThermalSystem/Front Side HXs/Radiator/Heat Capacity Rate ==
  AirMassFlw : Inport
  CpAir : Inport  Port=2
  CoolMFlw : Inport  Port=3
  CpCool : Inport  Port=4
  Divide2 : Product  Inputs=*/  RndMeth=Zero  SaturateOnIntegerOverflow=on
  Min : MinMax  Function=max  Inputs=2
  Min1 : MinMax  Inputs=2
  Product : Product
  Product1 : Product
  div0protect - abs poly2 : autolibutils/div0protect - abs poly  thresh=.001  aMode=1
  Cair : Outport
  Cmin : Outport  Port=2
  Cratio : Outport  Port=3
  Cmax : Outport  Port=4
  Ccool : Outport  Port=5
  wires:
  Product1/1 -> Ccool/1, [Ccool], Min/2
  [Ccool] -> Min1/2  "Ccool"
  Min/1 -> Cmax/1, div0protect - abs poly2/1  "Cmax"
  CpAir/1 -> Product/2
  Min1/1 -> Cmin/1, Divide2/1
  div0protect - abs poly2/1 -> Divide2/2
  Product/1 -> Cair/1, Min1/1, Min/1
  Divide2/1 -> Cratio/1
  CpCool/1 -> Product1/2
  AirMassFlw/1 -> Product/1
  CoolMFlw/1 -> Product1/1

== system ElectricalThermalSystem/Front Side HXs/Radiator/NTU and Dimensions ==
  FluidTemp1 : Inport
  MassFlow1 : Inport  Port=2
  MassFlow2 : Inport  Port=3
  FluidTemp2 : Inport  Port=4
  Cmin : Inport  Port=5
  Add : Sum
  Bias : Bias  Bias=1  SaturateOnIntegerOverflow=off
  Constant : Constant  Value=NTubes  SampleTime=-1
  Constant1 : Constant  Value=DhCool  SampleTime=-1
  Constant2 : Constant  Value=RadWid  SampleTime=-1
  Constant4 : Constant  Value=DhAir  SampleTime=-1
  Constant6 : Constant  Value=RadLen  SampleTime=-1
  Constant7 : Constant  Value=AcCool  SampleTime=-1
  Constant8 : Constant  Value=AcAir  SampleTime=-1
  Divide : Product  Inputs=*/
  Divide1 : Product  Inputs=*/
  Divide3 : Product  Inputs=*/
  Gain : Gain  Gain=PlntThrRadAirArea
  Gain1 : Gain  Gain=PlntThrRadAirArea
  HTC Estimator Air : Subsystem
      mask DialogControl Control1 Prompt: Convective Heat Transfer Coefficient (HTC) Estimator
      mask DialogControl Container2 Prompt: Description
      mask DialogControl Control2 Prompt: Assumes turbulent flow through a tube.
      mask DialogControl Control3 Prompt: The Nusselt number (NuD) is calculated with empirical formulas depending on 1/DoL.
      mask DialogControl Control4 Prompt: Where:
      mask DialogControl Control5 Prompt: DoL = hydraulic diameter / tube length
      mask DialogControl Control6 Prompt: When 1/DoL >= 400: NuD = 0.023*ReD^0.8*Pr^0.33
      mask DialogControl Control7 Prompt: Where:
      mask DialogControl Control8 Prompt: Pr: Prandtl number, out of 1D LUT depending on fluid temperature
      mask DialogControl Control9 Prompt: ReD: Reynolds number, calculated. ReD = mdot*hdia/(Ac*aVsc)
      mask DialogControl Control10 Prompt: Where:
      mask DialogControl Control11 Prompt: mdot: mass flow
      mask DialogControl Control12 Prompt: hdia: hydraulic diameter
      mask DialogControl Control13 Prompt: Ac: cross section area
      mask DialogControl Control14 Prompt: aVsc: absolute viscosity, out of 1D LUT depending on fluid temperature
      mask DialogControl Control15 Prompt: When 1/DoL < 400: NuD = 0.36*ReD^0.8*Pr^0.33*DoL^0.055
      mask DialogControl Control16 Prompt: Finally, HTC = k*NuD/hdia
      mask DialogControl Control17 Prompt: Where:
      mask DialogControl Control18 Prompt: k: thermal conductivity, out of 1D LUT depending on fluid temperature
  HTC Estimator Coolant : Subsystem
      mask DialogControl Control1 Prompt: Convective Heat Transfer Coefficient (HTC) Estimator
      mask DialogControl Container2 Prompt: Description
      mask DialogControl Control2 Prompt: Assumes turbulent flow through a tube.
      mask DialogControl Control3 Prompt: The Nusselt number (NuD) is calculated with empirical formulas depending on 1/DoL.
      mask DialogControl Control4 Prompt: Where:
      mask DialogControl Control5 Prompt: DoL = hydraulic diameter / tube length
      mask DialogControl Control6 Prompt: When 1/DoL >= 400: NuD = 0.023*ReD^0.8*Pr^0.33
      mask DialogControl Control7 Prompt: Where:
      mask DialogControl Control8 Prompt: Pr: Prandtl number, out of 1D LUT depending on fluid temperature
      mask DialogControl Control9 Prompt: ReD: Reynolds number, calculated. ReD = mdot*hdia/(Ac*aVsc)
      mask DialogControl Control10 Prompt: Where:
      mask DialogControl Control11 Prompt: mdot: mass flow
      mask DialogControl Control12 Prompt: hdia: hydraulic diameter
      mask DialogControl Control13 Prompt: Ac: cross section area
      mask DialogControl Control14 Prompt: aVsc: absolute viscosity, out of 1D LUT depending on fluid temperature
      mask DialogControl Control15 Prompt: When 1/DoL < 400: NuD = 0.36*ReD^0.8*Pr^0.33*DoL^0.055
      mask DialogControl Control16 Prompt: Finally, HTC = k*NuD/hdia
      mask DialogControl Control17 Prompt: Where:
      mask DialogControl Control18 Prompt: k: thermal conductivity, out of 1D LUT depending on fluid temperature
  Math Function : Math  Operator=reciprocal
  Math Function1 : Math  Operator=reciprocal
  Math Function2 : Math  Operator=reciprocal
  div0protect - abs poly{1..5} (5 alike) : autolibutils/div0protect - abs poly  thresh=.001  aMode=1
  NTU : Outport
  wires:
  Constant2/1 -> HTC Estimator Air/5(TubLen)
  HTC Estimator Coolant/1(HTC) -> Gain/1
  Constant6/1 -> HTC Estimator Coolant/5(TubLen)
  Constant/1 -> div0protect - abs poly1/1, Bias/1
  MassFlow1/1 -> Divide/1
  Bias/1 -> Divide1/2
  FluidTemp2/1 -> HTC Estimator Air/1(FluidTemp)
  Divide/1 -> HTC Estimator Coolant/2(MassFlow)
  FluidTemp1/1 -> HTC Estimator Coolant/1(FluidTemp)
  Constant7/1 -> HTC Estimator Coolant/3(CrossA)
  Divide1/1 -> HTC Estimator Air/2(MassFlow)
  Constant8/1 -> HTC Estimator Air/3(CrossA)
  HTC Estimator Air/1(HTC) -> Gain1/1
  Constant1/1 -> HTC Estimator Coolant/4(HydDia)
  Constant4/1 -> HTC Estimator Air/4(HydDia)
  MassFlow2/1 -> Divide1/1
  Divide3/1 -> NTU/1
  div0protect - abs poly3/1 -> Divide3/2
  Cmin/1 -> div0protect - abs poly3/1
  div0protect - abs poly1/1 -> Divide/2
  Math Function2/1 -> Divide3/1
  div0protect - abs poly5/1 -> Math Function2/1
  Add/1 -> div0protect - abs poly5/1
  div0protect - abs poly4/1 -> Math Function1/1
  Gain1/1 -> div0protect - abs poly4/1
  Gain/1 -> div0protect - abs poly2/1
  div0protect - abs poly2/1 -> Math Function/1
  Math Function/1 -> Add/1
  Math Function1/1 -> Add/2

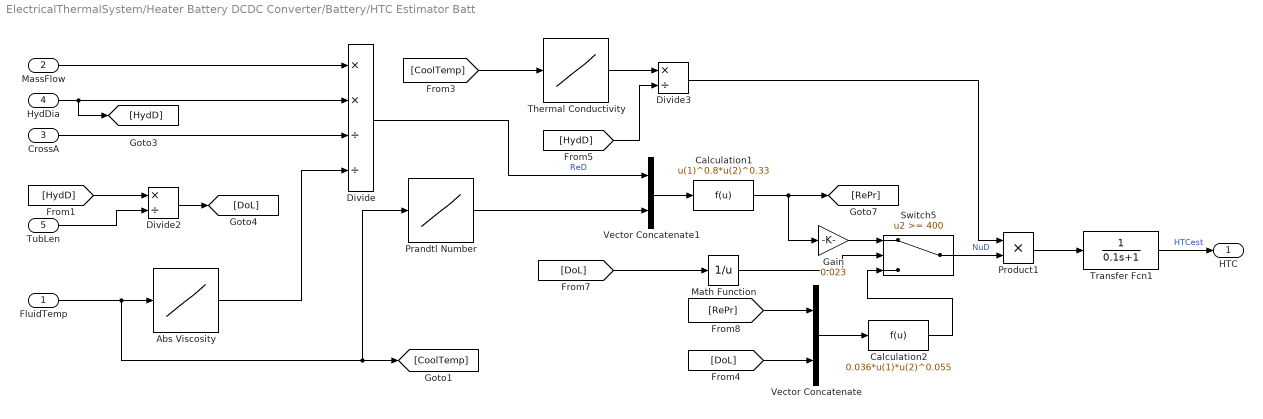
== system ElectricalThermalSystem/Heater Battery DCDC Converter/Battery/HTC Estimator Batt ==
  FluidTemp : Inport
  MassFlow : Inport  Port=2
  CrossA : Inport  Port=3  OutMin=eps
  HydDia : Inport  Port=4
  TubLen : Inport  Port=5
  Abs Viscosity : Lookup_n-D  NumberOfTableDimensions=1  BreakpointsForDimension1=PlntThrCoolCpBpt  Table=PlntThrCoolVisc  ExtrapMethod=Clip  UseLastTableValue=on  InternalRulePriority=Speed  RndMeth=Simplest
  Calculation1 : Fcn  Expr=u(1)^0.8*u(2)^0.33
  Calculation2 : Fcn  Expr=0.036*u(1)*u(2)^0.055
  Divide : Product  Inputs=**//
  Divide2 : Product  Inputs=*/
  Divide3 : Product  Inputs=*/
  Gain : Gain  Gain=0.023
  Math Function : Math  Operator=reciprocal
  Prandtl Number : Lookup_n-D  NumberOfTableDimensions=1  BreakpointsForDimension1=PlntThrCoolCpBpt  Table=PlntThrCoolPrand  ExtrapMethod=Clip  UseLastTableValue=on  InternalRulePriority=Speed  RndMeth=Simplest
  Product1 : Product
  Switch5 : Switch  Threshold=400  SaturateOnIntegerOverflow=off  InputSameDT=off
  Thermal Conductivity : Lookup_n-D  NumberOfTableDimensions=1  BreakpointsForDimension1=PlntThrCoolCpBpt  Table=PlntThrCoolCond  ExtrapMethod=Clip  UseLastTableValue=on  InternalRulePriority=Speed  RndMeth=Simplest
  Transfer Fcn1 : TransferFcn  Denominator=[0.1 1]
  Vector Concatenate : Concatenate
  Vector Concatenate1 : Concatenate
  HTC : Outport
  wires:
  Transfer Fcn1/1 -> HTC/1  "HTCest"
  FluidTemp/1 -> Prandtl Number/1, [CoolTemp], Abs Viscosity/1
  [CoolTemp] -> Thermal Conductivity/1
  MassFlow/1 -> Divide/1
  HydDia/1 -> [HydD], Divide/2
  CrossA/1 -> Divide/3
  [HydD] -> Divide2/1
  TubLen/1 -> Divide2/2
  Divide2/1 -> [DoL]
  Abs Viscosity/1 -> Divide/4
  Divide/1 -> Vector Concatenate1/1  "ReD"
  Prandtl Number/1 -> Vector Concatenate1/2
  Vector Concatenate1/1 -> Calculation1/1
  [DoL] -> Math Function/1
  Math Function/1 -> Switch5/2
  Thermal Conductivity/1 -> Divide3/1
  [HydD] -> Divide3/2
  Divide3/1 -> Product1/1
  Gain/1 -> Switch5/1
  Calculation1/1 -> [RePr], Gain/1
  [RePr] -> Vector Concatenate/1
  [DoL] -> Vector Concatenate/2
  Vector Concatenate/1 -> Calculation2/1
  Calculation2/1 -> Switch5/3
  Switch5/1 -> Product1/2  "NuD"
  Product1/1 -> Transfer Fcn1/1

== system ElectricalThermalSystem/Heater Battery DCDC Converter/Battery/Heat-flow Rate ==
  HTC : Inport
  JacHtArea : Inport  Port=2
  BattTemp : Inport  Port=3
  CoolBlkTemp : Inport  Port=4
  Product2 : Product  Inputs=3
  Subtract1 : Sum  Inputs=+-
  Qbatt : Outport
  wires:
  HTC/1 -> Product2/1
  Subtract1/1 -> Product2/3
  JacHtArea/1 -> Product2/2
  CoolBlkTemp/1 -> Subtract1/2
  Product2/1 -> Qbatt/1
  BattTemp/1 -> Subtract1/1

== system ElectricalThermalSystem/Heater Battery DCDC Converter/Battery Heater/LPF with IC3 ==
  u : Inport
  Cont LPF IC : autolibutils/Cont LPF IC  wc=wc  aMode=1  dataType=off
  Initial Condition : Constant  Value=InitCond  SampleTime=-1
  y : Outport
  wires:
  Initial Condition/1 -> Cont LPF IC/2
  u/1 -> Cont LPF IC/1
  Cont LPF IC/1 -> y/1

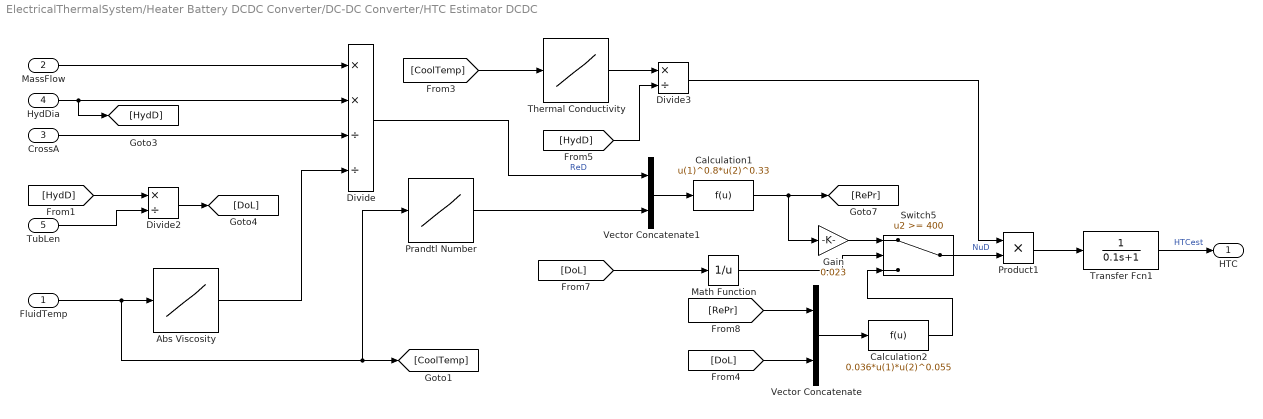
== system ElectricalThermalSystem/Heater Battery DCDC Converter/DC-DC Converter/HTC Estimator DCDC ==
  FluidTemp : Inport
  MassFlow : Inport  Port=2
  CrossA : Inport  Port=3  OutMin=eps
  HydDia : Inport  Port=4
  TubLen : Inport  Port=5
  Abs Viscosity : Lookup_n-D  NumberOfTableDimensions=1  BreakpointsForDimension1=PlntThrCoolCpBpt  Table=PlntThrCoolVisc  ExtrapMethod=Clip  UseLastTableValue=on  InternalRulePriority=Speed  RndMeth=Simplest
  Calculation1 : Fcn  Expr=u(1)^0.8*u(2)^0.33
  Calculation2 : Fcn  Expr=0.036*u(1)*u(2)^0.055
  Divide : Product  Inputs=**//
  Divide2 : Product  Inputs=*/
  Divide3 : Product  Inputs=*/
  Gain : Gain  Gain=0.023
  Math Function : Math  Operator=reciprocal
  Prandtl Number : Lookup_n-D  NumberOfTableDimensions=1  BreakpointsForDimension1=PlntThrCoolCpBpt  Table=PlntThrCoolPrand  ExtrapMethod=Clip  UseLastTableValue=on  InternalRulePriority=Speed  RndMeth=Simplest
  Product1 : Product
  Switch5 : Switch  Threshold=400  SaturateOnIntegerOverflow=off  InputSameDT=off
  Thermal Conductivity : Lookup_n-D  NumberOfTableDimensions=1  BreakpointsForDimension1=PlntThrCoolCpBpt  Table=PlntThrCoolCond  ExtrapMethod=Clip  UseLastTableValue=on  InternalRulePriority=Speed  RndMeth=Simplest
  Transfer Fcn1 : TransferFcn  Denominator=[0.1 1]
  Vector Concatenate : Concatenate
  Vector Concatenate1 : Concatenate
  HTC : Outport
  wires:
  Transfer Fcn1/1 -> HTC/1  "HTCest"
  FluidTemp/1 -> Prandtl Number/1, [CoolTemp], Abs Viscosity/1
  [CoolTemp] -> Thermal Conductivity/1
  MassFlow/1 -> Divide/1
  HydDia/1 -> [HydD], Divide/2
  CrossA/1 -> Divide/3
  [HydD] -> Divide2/1
  TubLen/1 -> Divide2/2
  Divide2/1 -> [DoL]
  Abs Viscosity/1 -> Divide/4
  Divide/1 -> Vector Concatenate1/1  "ReD"
  Prandtl Number/1 -> Vector Concatenate1/2
  Vector Concatenate1/1 -> Calculation1/1
  [DoL] -> Math Function/1
  Math Function/1 -> Switch5/2
  Thermal Conductivity/1 -> Divide3/1
  [HydD] -> Divide3/2
  Divide3/1 -> Product1/1
  Gain/1 -> Switch5/1
  Calculation1/1 -> [RePr], Gain/1
  [RePr] -> Vector Concatenate/1
  [DoL] -> Vector Concatenate/2
  Vector Concatenate/1 -> Calculation2/1
  Calculation2/1 -> Switch5/3
  Switch5/1 -> Product1/2  "NuD"
  Product1/1 -> Transfer Fcn1/1

== system ElectricalThermalSystem/Heater Battery DCDC Converter/DC-DC Converter/Heat-flow Rate ==
  HTC : Inport
  PwrETemp : Inport  Port=2
  JacArea : Inport  Port=3
  CoolBlkTemp : Inport  Port=4
  Product1 : Product  Inputs=3
  Subtract : Sum  Inputs=+-
  Qpwre : Outport
  wires:
  JacArea/1 -> Product1/2
  Subtract/1 -> Product1/3
  PwrETemp/1 -> Subtract/1
  CoolBlkTemp/1 -> Subtract/2
  Product1/1 -> Qpwre/1
  HTC/1 -> Product1/1
